simulink model "PI_controller"  (R2020a)
settings: Solver=VariableStepAuto  StartTime=0.0  StopTime=10.0  RelTol=1e-3
undefined symbols (not defined in the file or in its folder): Ki, Kp, Ts
settings Model: OrderedModelArguments=off  Creator=NIKITA  LastModifiedBy=NIKITA

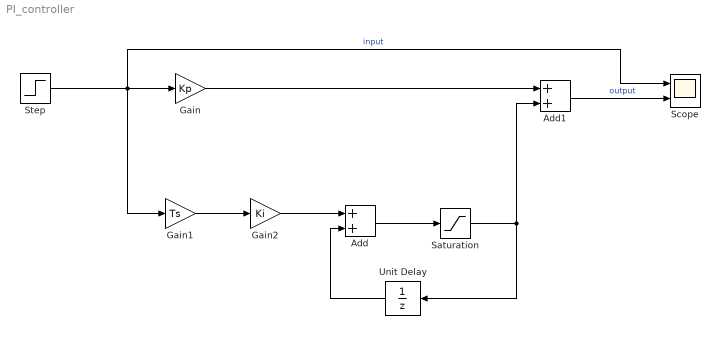
== system PI_controller ==
  Add : Sum
  Add1 : Sum
  Gain : Gain  Gain=Kp
  Gain1 : Gain  Gain=Ts
  Gain2 : Gain  Gain=Ki
  Saturation : Saturate  UpperLimit=1  LowerLimit=-1
  Scope : Scope  NumInputPorts=2
  Step : Step  SampleTime=Ts
  Unit Delay : UnitDelay  SampleTime=-1  HasFrameUpgradeWarning=on
  wires:
  Add/1 -> Saturation/1
  Saturation/1 -> Unit Delay/1, Add1/2
  Gain/1 -> Add1/1
  Gain1/1 -> Gain2/1
  Step/1 -> Scope/1, Gain1/1, Gain/1  "input"
  Unit Delay/1 -> Add/2
  Gain2/1 -> Add/1
  Add1/1 -> Scope/2  "output"
